simulink model "ExpCtrlXdirection"  (R2013a)
settings: Solver=ode45  StartTime=0.0  StopTime=5.0  RelTol=1e-3
undefined symbols (not defined in the file): modelXdirectionReal, TsReal, x0
libraries: mpt_sim x1
settings Model: Creator=root  LastModifiedBy=root

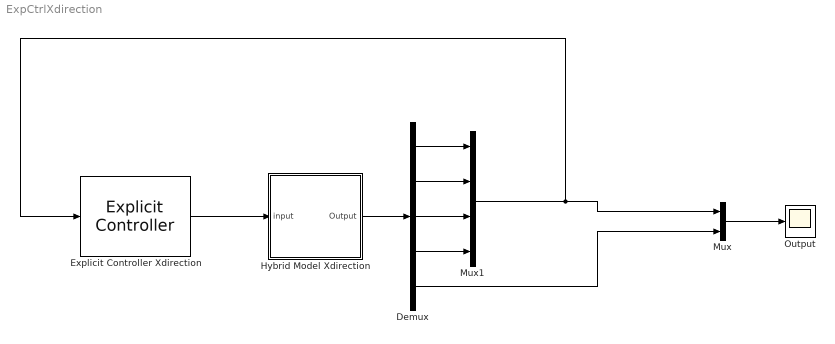
== system ExpCtrlXdirection ==
  Demux : Demux  Outputs=5
  Explicit Controller Xdirection : mpt_sim/Explicit Controller
      link override S-Function: FunctionName=mpt_getInput_sfunc_Xdirection
  Hybrid Model Xdirection : Subsystem
  Mux : Mux  Inputs=2
  Mux1 : Mux
  Output : Scope
      settings: YMin=-3.25  YMax=1.5
  wires:
  Explicit Controller Xdirection/1 -> Hybrid Model Xdirection/1(input)
  Mux/1 -> Output/1
  Demux/5 -> Mux/2
  Demux/3 -> Mux1/3
  Demux/4 -> Mux1/4
  Demux/1 -> Mux1/1
  Demux/2 -> Mux1/2
  Mux1/1 -> Explicit Controller Xdirection/1, Mux/1
  Hybrid Model Xdirection/1(Output) -> Demux/1

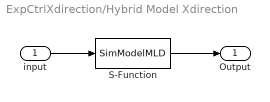
== system ExpCtrlXdirection/Hybrid Model Xdirection ==
  input : Inport
  S-Function : S-Function  FunctionName=SimModelMLD  Parameters=modelXdirectionReal,x0,TsReal  EnableBusSupport=off
  Output : Outport
  wires:
  input/1 -> S-Function/1
  S-Function/1 -> Output/1
